simulink model "ACC_Test_module"  (R2017b)
settings: Solver=FixedStepAuto  StartTime=0.0  StopTime=150  FixedStep=0.05  RelTol=1e-3
libraries: simulink x4, SimOneModule x3
settings Model: Creator=weinan  LastModifiedBy=xuliang
settings SolverCC: AlgebraicLoopSolver=LineSearch

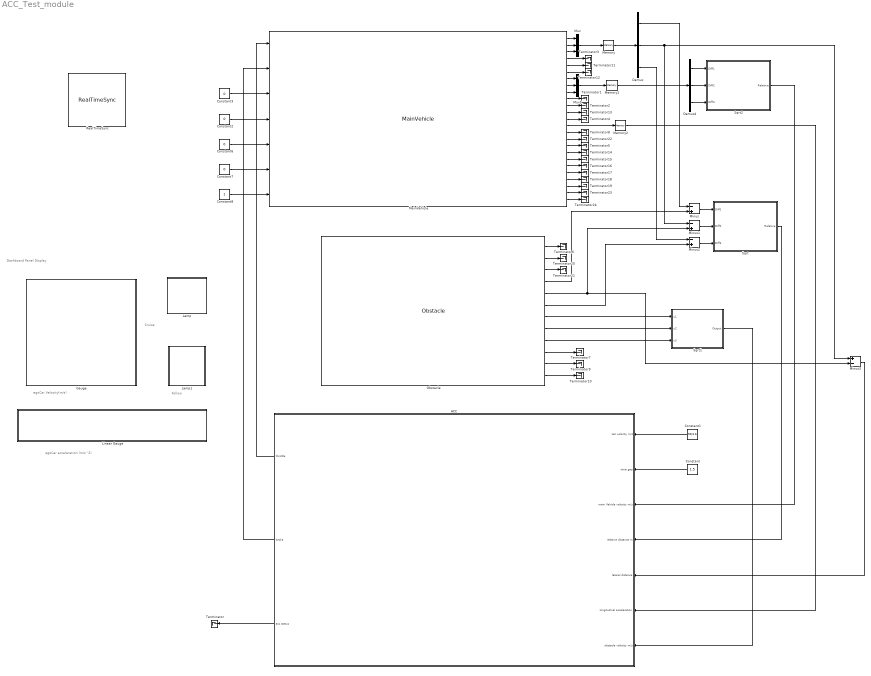
== system ACC_Test_module ==
  note: Cruise
  note: egoCar Velocity(m/s)
  note: Follow
  note: Dashboard Panel Display
  note: egoCar acceleration (m/s^2)
  "ACC " : Subsystem  mask(ACC){}
      mask help: ACC block
  Constant : Constant  Value=1.5  OutDataTypeStr=single
  Constant1 : Constant  Value=50/3.6  OutDataTypeStr=single
  Constant2 : Constant  Value=0  OutDataTypeStr=single
  Constant3 : Constant  Value=0  OutDataTypeStr=int32
  Constant6 : Constant  Value=0  OutDataTypeStr=boolean
  Constant7 : Constant  Value=0  OutDataTypeStr=boolean
  Constant8 : Constant  OutDataTypeStr=int32
  Demux : Demux  Outputs=3
  Demux4 : Demux  Outputs=3
  Gauge : Subsystem  DialogController=hmiCreateDDGDialog  IsWebBlock=on  mask(MWDashboardBlock){webBlockId=47d9afb7-ca15-4b52-9b06-8f3727cd5279, webBlockType=circulargauge, ShowInLibBrowser=on, ShowInitialText=on, HMISrcModelName=ACC_Test_module}
      mask prompts: webBlockId "WebBlock Id"; webBlockType "WebBlock Type"; HMISrcModelName "Source Model"
      mask help: SimulinkHMI:dialogs:CircularGaugeDialogDesc
      mask Help: helpview([docroot '/mapfiles/simulink.map'], 'hmi_gauge')
      mask Display:
      | if strcmp(get_param(bdroot(gcb),'BlockDiagramType'), 'library')
      |     image([(matlabroot) '/toolbox/simulink/hmi/icons/CircularGauge.png']);
      | end
  Lamp : Subsystem  DialogController=hmiCreateDDGDialog  IsWebBlock=on  mask(MWDashboardBlock){webBlockId=fddfa241-ada3-46a5-89fa-7b193cbd09ab, webBlockType=lamp, ShowInLibBrowser=on, ShowInitialText=on, HMISrcModelName=ACC_Test_module}
      mask prompts: webBlockId "WebBlock Id"; webBlockType "WebBlock Type"; HMISrcModelName "Source Model"
      mask help: Display a color that reflects an input value.
      mask Help: helpview([docroot '/mapfiles/simulink.map'], 'hmi_lamp')
      mask Display:
      | if strcmp(get_param(bdroot(gcb),'BlockDiagramType'),'library')
      |  image([(matlabroot) '/toolbox/simulink/hmi/icons/Lamp.png'])
      | end
  Lamp1 : Subsystem  DialogController=hmiCreateDDGDialog  IsWebBlock=on  mask(MWDashboardBlock){webBlockId=92ae66d2-b6c3-43d2-a72d-fb865ca14b34, webBlockType=lamp, ShowInLibBrowser=on, ShowInitialText=on, HMISrcModelName=ACC_Test_module}
      mask prompts: webBlockId "WebBlock Id"; webBlockType "WebBlock Type"; HMISrcModelName "Source Model"
      mask help: Display a color that reflects an input value.
      mask Help: helpview([docroot '/mapfiles/simulink.map'], 'hmi_lamp')
      mask Display:
      | if strcmp(get_param(bdroot(gcb),'BlockDiagramType'),'library')
      |  image([(matlabroot) '/toolbox/simulink/hmi/icons/Lamp.png'])
      | end
  Linear Gauge : Subsystem  DialogController=hmiCreateDDGDialog  IsWebBlock=on  mask(MWDashboardBlock){webBlockId=739a4254-edef-4805-a255-418ead3e1f6d, webBlockType=lineargauge, ShowInLibBrowser=on, ShowInitialText=on, HMISrcModelName=ACC_Test_module}
      mask prompts: webBlockId "WebBlock Id"; webBlockType "WebBlock Type"; HMISrcModelName "Source Model"
      mask help: SimulinkHMI:dialogs:LinearGaugeDialogDesc
      mask Help: helpview([docroot '/mapfiles/simulink.map'], 'hmi_linear_gauge')
      mask Display:
      | if strcmp(get_param(bdroot(gcb),'BlockDiagramType'), 'library')
      |     image([(matlabroot) '/toolbox/simulink/hmi/icons/LinearGauge.png']);
      | end
  MainVehicle : SimOneModule/MainVehicle
  Memory : Memory
  Memory1 : Memory
  Memory2 : Memory
  Minus : Sum  Inputs=-+
  Minus1 : Sum  Inputs=-+
  Minus2 : Sum  Inputs=-+
  Minus3 : Sum  Inputs=+-
  Mux : Mux  Inputs=3
  Mux1 : Mux  Inputs=3
  Obstacle : SimOneModule/Obstacle  MaxObstacleNum=10  ObstacleId=1
  RealTimeSync : SimOneModule/RealTimeSync
  "Sqrt " : Subsystem  mask(Sqrt){}
      mask help: Square root of the sum of squared inputs
  Sqrt1 : Subsystem  mask(Sqrt){}
      mask help: Square root of the sum of squared inputs
  Sqrt2 : Subsystem  mask(Sqrt){}
      mask help: Square root of the sum of squared inputs
  Terminator{,1..24} (25 alike) : Terminator
  wires:
  Constant8/1 -> MainVehicle/7
  Constant7/1 -> MainVehicle/6
  Constant6/1 -> MainVehicle/5
  Constant/1 -> "ACC "/2(time gap)
  Constant1/1 -> "ACC "/1(set velocity m/s)
  Mux/1 -> Memory/1
  "Sqrt "/1(Relative) -> "ACC "/4(relative distance m)
  Minus3/1 -> "ACC "/5(lateral distance)
  "ACC "/3(acc status) -> Terminator/1
  Memory/1 -> Demux/1
  Memory1/1 -> Demux4/1
  MainVehicle/11 -> Terminator2/1
  Minus/1 -> "Sqrt "/1(Diff1)
  Minus1/1 -> "Sqrt "/2(Diff2)
  Minus2/1 -> "Sqrt "/3(Diff3)
  Demux/1 -> Minus/1
  Demux/2 -> Minus3/1, Minus1/1
  Demux/3 -> Minus2/1
  Obstacle/4 -> Minus/2
  Obstacle/5 -> Minus3/2, Minus1/2
  Obstacle/6 -> Minus2/2
  Demux4/1 -> Sqrt2/1(Diff1)
  Demux4/2 -> Sqrt2/2(Diff2)
  Demux4/3 -> Sqrt2/3(Diff3)
  Sqrt2/1(Relative) -> "ACC "/3(main Vehicle velocity m/s)
  Sqrt1/1(Output) -> "ACC "/7(obstacle velocity m/s)
  Constant2/1 -> MainVehicle/4
  Memory2/1 -> "ACC "/6(longitudinal acceleration)
  MainVehicle/4 -> Terminator3/1
  Obstacle/10 -> Terminator7/1
  Obstacle/11 -> Terminator9/1
  Obstacle/12 -> Terminator10/1
  MainVehicle/2 -> Mux/2
  MainVehicle/1 -> Mux/1
  MainVehicle/3 -> Mux/3
  MainVehicle/5 -> Terminator11/1
  MainVehicle/6 -> Terminator12/1
  Mux1/1 -> Memory1/1
  MainVehicle/10 -> Terminator1/1
  MainVehicle/12 -> Terminator13/1
  MainVehicle/13 -> Terminator4/1
  MainVehicle/17 -> Terminator5/1
  MainVehicle/18 -> Terminator14/1
  MainVehicle/19 -> Terminator15/1
  MainVehicle/20 -> Terminator16/1
  MainVehicle/21 -> Terminator17/1
  MainVehicle/22 -> Terminator18/1
  MainVehicle/23 -> Terminator19/1
  Obstacle/1 -> Terminator6/1
  Obstacle/2 -> Terminator20/1
  Obstacle/3 -> Terminator21/1
  MainVehicle/14 -> Memory2/1
  MainVehicle/15 -> Terminator8/1
  MainVehicle/16 -> Terminator22/1
  "ACC "/1(throttle) -> MainVehicle/1
  "ACC "/2(brake) -> MainVehicle/2
  Obstacle/8 -> Sqrt1/2(u2)
  MainVehicle/8 -> Mux1/2
  Obstacle/9 -> Sqrt1/3(u3)
  MainVehicle/7 -> Mux1/1
  Obstacle/7 -> Sqrt1/1(u1)
  MainVehicle/9 -> Mux1/3
  MainVehicle/24 -> Terminator23/1
  MainVehicle/25 -> Terminator24/1
  Constant3/1 -> MainVehicle/3

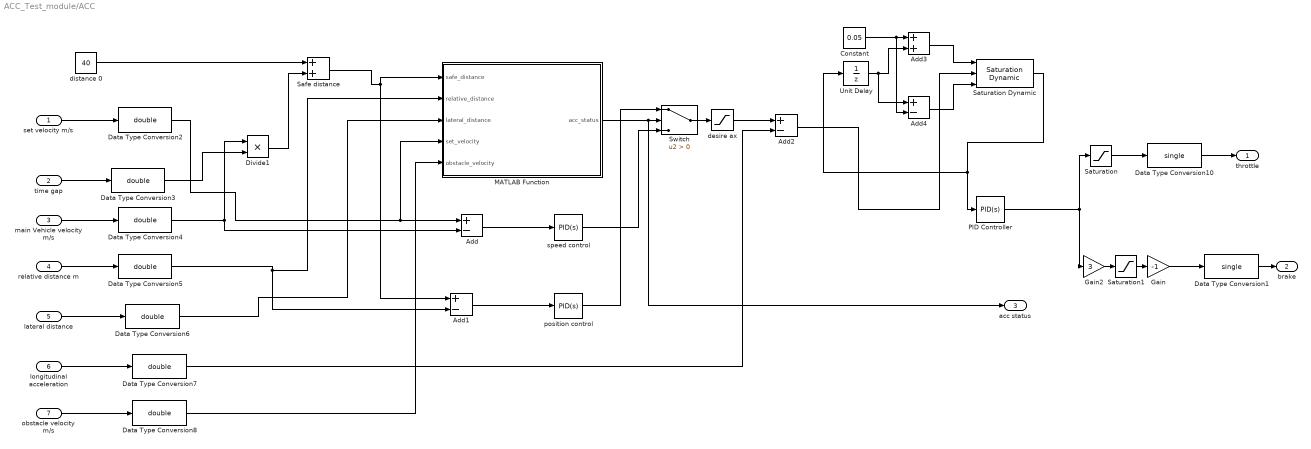
== system ACC_Test_module/ACC  ==
  set velocity m/s : Inport
  time gap : Inport  Port=2
  main Vehicle velocity m/s : Inport  Port=3
  relative distance m : Inport  Port=4
  lateral distance : Inport  Port=5
  longitudinal acceleration : Inport  Port=6
  obstacle velocity m/s : Inport  Port=7
  Add{,1..2,4} (4 alike) : Sum  Inputs=+-
  Add3 : Sum
  Constant : Constant  Value=0.05  OutDataTypeStr=double
  Data Type Conversion1 : DataTypeConversion  OutDataTypeStr=single
  Data Type Conversion10 : DataTypeConversion  OutDataTypeStr=single
  Data Type Conversion{2..8} (7 alike) : DataTypeConversion  OutDataTypeStr=double
  Divide1 : Product  Inputs=**
  Gain : Gain  Gain=-1
  Gain2 : Gain  Gain=3
  MATLAB Function : MATLAB Function  TreatAsAtomicUnit=on
  PID Controller : simulink/Continuous/PID Controller  Controller=PID  TimeDomain=Continuous-time  SampleTime=-1  IntegratorMethod=Forward Euler  FilterMethod=Forward Euler  Form=Parallel  UseFilter=on  ControllerParametersSource=internal  P=0.2  I=0  D=0  N=100  InitialConditionSource=internal  InitialConditionForIntegrator=0  InitialConditionForFilter=0  ExternalReset=none  LimitOutput=off  UpperSaturationLimit=inf  LowerSaturationLimit=-inf  LinearizeAsGain=on  AntiWindupMode=none  Kb=1  TrackingMode=off  Kt=1  PParamMin=[]  PParamMax=[]  IParamMin=[]  IParamMax=[]  DParamMin=[]  DParamMax=[]  NParamMin=[]  NParamMax=[]  KbParamMin=[]  KbParamMax=[]  KtParamMin=[]  KtParamMax=[]  POutMin=[]  POutMax=[]  IOutMin=[]  IOutMax=[]  DOutMin=[]  DOutMax=[]  NOutMin=[]  NOutMax=[]  KbOutMin=[]  KbOutMax=[]  KtOutMin=[]  KtOutMax=[]  IntegratorOutMin=[]  IntegratorOutMax=[]  FilterOutMin=[]  FilterOutMax=[]  SumOutMin=[]  SumOutMax=[]  SumI1OutMin=[]  SumI1OutMax=[]  SumI2OutMin=[]  SumI2OutMax=[]  SumI3OutMin=[]  SumI3OutMax=[]  SumDOutMin=[]  SumDOutMax=[]  SaturationOutMin=[]  SaturationOutMax=[]  IntegratorContinuousStateAttributes=''  IntegratorStateMustResolveToSignalObject=off  IntegratorRTWStateStorageClass=Auto  FilterContinuousStateAttributes=''  FilterStateMustResolveToSignalObject=off  FilterRTWStateStorageClass=Auto  DifferentiatorICPrevScaledInput=0  DifferentiatorOutMin=[]  DifferentiatorOutMax=[]  FilterDiffOutCoefMin=[]  FilterDiffOutCoefMax=[]  SumDenOutMin=[]  SumDenOutMax=[]  SumNumOutMin=[]  SumNumOutMax=[]  ReciprocalOutMin=[]  ReciprocalOutMax=[]  DivideOutMin=[]  DivideOutMax=[]  TunerSelectOption=Transfer Function Based (PID Tuner App)
  Safe distance : Sum
  Saturation : Saturate  UpperLimit=1  LowerLimit=0
  Saturation Dynamic : simulink/Discontinuities/Saturation Dynamic  OutMin=[]  OutMax=[]  OutDataTypeStr=Inherit: Same as second input  OutDataType=fixdt(1, 16)  OutScaling=2^-10  DoSatur=off
  Saturation1 : Saturate  UpperLimit=0  LowerLimit=-1
  Switch : Switch  Criteria=u2 > Threshold
  Unit Delay : UnitDelay  SampleTime=-1
  desire ax : Saturate  UpperLimit=8  LowerLimit=-3
  distance 0 : Constant  Value=40  OutDataTypeStr=double
  position control : simulink/Continuous/PID Controller  Controller=PID  TimeDomain=Continuous-time  SampleTime=-1  IntegratorMethod=Forward Euler  FilterMethod=Forward Euler  Form=Parallel  UseFilter=on  ControllerParametersSource=internal  P=-0.03  I=0  D=0  N=100  InitialConditionSource=internal  InitialConditionForIntegrator=0  InitialConditionForFilter=0  ExternalReset=none  LimitOutput=off  UpperSaturationLimit=inf  LowerSaturationLimit=-inf  LinearizeAsGain=on  AntiWindupMode=none  Kb=1  TrackingMode=off  Kt=1  PParamMin=[]  PParamMax=[]  IParamMin=[]  IParamMax=[]  DParamMin=[]  DParamMax=[]  NParamMin=[]  NParamMax=[]  KbParamMin=[]  KbParamMax=[]  KtParamMin=[]  KtParamMax=[]  POutMin=[]  POutMax=[]  IOutMin=[]  IOutMax=[]  DOutMin=[]  DOutMax=[]  NOutMin=[]  NOutMax=[]  KbOutMin=[]  KbOutMax=[]  KtOutMin=[]  KtOutMax=[]  IntegratorOutMin=[]  IntegratorOutMax=[]  FilterOutMin=[]  FilterOutMax=[]  SumOutMin=[]  SumOutMax=[]  SumI1OutMin=[]  SumI1OutMax=[]  SumI2OutMin=[]  SumI2OutMax=[]  SumI3OutMin=[]  SumI3OutMax=[]  SumDOutMin=[]  SumDOutMax=[]  SaturationOutMin=[]  SaturationOutMax=[]  IntegratorContinuousStateAttributes=''  IntegratorStateMustResolveToSignalObject=off  IntegratorRTWStateStorageClass=Auto  FilterContinuousStateAttributes=''  FilterStateMustResolveToSignalObject=off  FilterRTWStateStorageClass=Auto  DifferentiatorICPrevScaledInput=0  DifferentiatorOutMin=[]  DifferentiatorOutMax=[]  FilterDiffOutCoefMin=[]  FilterDiffOutCoefMax=[]  SumDenOutMin=[]  SumDenOutMax=[]  SumNumOutMin=[]  SumNumOutMax=[]  ReciprocalOutMin=[]  ReciprocalOutMax=[]  DivideOutMin=[]  DivideOutMax=[]  TunerSelectOption=Transfer Function Based (PID Tuner App)
  speed control : simulink/Continuous/PID Controller  Controller=PID  TimeDomain=Continuous-time  SampleTime=-1  IntegratorMethod=Forward Euler  FilterMethod=Forward Euler  Form=Parallel  UseFilter=on  ControllerParametersSource=internal  P=0.6  I=0  D=0  N=100  InitialConditionSource=internal  InitialConditionForIntegrator=0  InitialConditionForFilter=0  ExternalReset=none  LimitOutput=off  UpperSaturationLimit=inf  LowerSaturationLimit=-inf  LinearizeAsGain=on  AntiWindupMode=none  Kb=1  TrackingMode=off  Kt=1  PParamMin=[]  PParamMax=[]  IParamMin=[]  IParamMax=[]  DParamMin=[]  DParamMax=[]  NParamMin=[]  NParamMax=[]  KbParamMin=[]  KbParamMax=[]  KtParamMin=[]  KtParamMax=[]  POutMin=[]  POutMax=[]  IOutMin=[]  IOutMax=[]  DOutMin=[]  DOutMax=[]  NOutMin=[]  NOutMax=[]  KbOutMin=[]  KbOutMax=[]  KtOutMin=[]  KtOutMax=[]  IntegratorOutMin=[]  IntegratorOutMax=[]  FilterOutMin=[]  FilterOutMax=[]  SumOutMin=[]  SumOutMax=[]  SumI1OutMin=[]  SumI1OutMax=[]  SumI2OutMin=[]  SumI2OutMax=[]  SumI3OutMin=[]  SumI3OutMax=[]  SumDOutMin=[]  SumDOutMax=[]  SaturationOutMin=[]  SaturationOutMax=[]  IntegratorContinuousStateAttributes=''  IntegratorStateMustResolveToSignalObject=off  IntegratorRTWStateStorageClass=Auto  FilterContinuousStateAttributes=''  FilterStateMustResolveToSignalObject=off  FilterRTWStateStorageClass=Auto  DifferentiatorICPrevScaledInput=0  DifferentiatorOutMin=[]  DifferentiatorOutMax=[]  FilterDiffOutCoefMin=[]  FilterDiffOutCoefMax=[]  SumDenOutMin=[]  SumDenOutMax=[]  SumNumOutMin=[]  SumNumOutMax=[]  ReciprocalOutMin=[]  ReciprocalOutMax=[]  DivideOutMin=[]  DivideOutMax=[]  TunerSelectOption=Transfer Function Based (PID Tuner App)
  throttle : Outport
  brake : Outport  Port=2
  acc status : Outport  Port=3
  wires:
  time gap/1 -> Data Type Conversion3/1
  Divide1/1 -> Safe distance/2
  Safe distance/1 -> Add1/1, MATLAB Function/1(safe_distance)
  relative distance m/1 -> Data Type Conversion5/1
  lateral distance/1 -> Data Type Conversion6/1
  main Vehicle velocity m/s/1 -> Data Type Conversion4/1
  set velocity m/s/1 -> Data Type Conversion2/1
  Add/1 -> speed control/1
  obstacle velocity m/s/1 -> Data Type Conversion8/1
  Add1/1 -> position control/1
  speed control/1 -> Switch/3
  position control/1 -> Switch/1
  Switch/1 -> desire ax/1
  desire ax/1 -> Add2/1
  longitudinal acceleration/1 -> Data Type Conversion7/1
  Saturation/1 -> Data Type Conversion10/1
  Saturation1/1 -> Gain/1
  Gain/1 -> Data Type Conversion1/1
  Gain2/1 -> Saturation1/1
  Constant/1 -> Add4/2, Add3/1
  Unit Delay/1 -> Add4/1, Add3/2
  Add3/1 -> Saturation Dynamic/1
  Add4/1 -> Saturation Dynamic/3
  Add2/1 -> Saturation Dynamic/2
  Saturation Dynamic/1 -> Unit Delay/1, PID Controller/1
  PID Controller/1 -> Saturation/1, Gain2/1
  distance 0/1 -> Safe distance/1
  Data Type Conversion2/1 -> MATLAB Function/4(set_velocity), Add/1
  Data Type Conversion3/1 -> Divide1/2
  Data Type Conversion4/1 -> Add/2, Divide1/1
  Data Type Conversion5/1 -> Add1/2, MATLAB Function/2(relative_distance)
  Data Type Conversion6/1 -> MATLAB Function/3(lateral_distance)
  Data Type Conversion7/1 -> Add2/2
  Data Type Conversion8/1 -> MATLAB Function/5(obstacle_velocity)
  MATLAB Function/1(acc_status) -> acc status/1, Switch/2
  Data Type Conversion1/1 -> brake/1
  Data Type Conversion10/1 -> throttle/1

== system ACC_Test_module/Gauge ==

== system ACC_Test_module/Lamp ==

== system ACC_Test_module/Lamp1 ==

== system ACC_Test_module/Linear Gauge ==

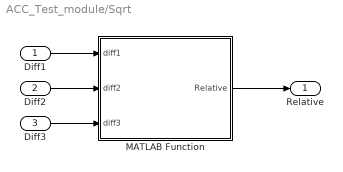
== system ACC_Test_module/Sqrt  ==
  Diff1 : Inport
  Diff2 : Inport  Port=2
  Diff3 : Inport  Port=3
  MATLAB Function : MATLAB Function  TreatAsAtomicUnit=on
  Relative : Outport
  wires:
  Diff1/1 -> MATLAB Function/1(diff1)
  MATLAB Function/1(Relative) -> Relative/1
  Diff2/1 -> MATLAB Function/2(diff2)
  Diff3/1 -> MATLAB Function/3(diff3)

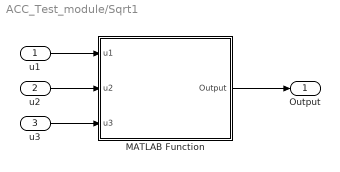
== system ACC_Test_module/Sqrt1 ==
  u1 : Inport
  u2 : Inport  Port=2
  u3 : Inport  Port=3
  MATLAB Function : MATLAB Function  TreatAsAtomicUnit=on
  Output : Outport
  wires:
  u1/1 -> MATLAB Function/1(u1)
  MATLAB Function/1(Output) -> Output/1
  u2/1 -> MATLAB Function/2(u2)
  u3/1 -> MATLAB Function/3(u3)

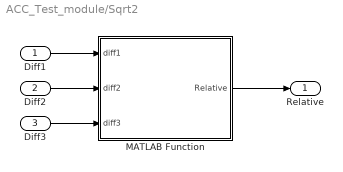
== system ACC_Test_module/Sqrt2 ==
  Diff1 : Inport
  Diff2 : Inport  Port=2
  Diff3 : Inport  Port=3
  MATLAB Function : MATLAB Function  TreatAsAtomicUnit=on
  Relative : Outport
  wires:
  Diff1/1 -> MATLAB Function/1(diff1)
  MATLAB Function/1(Relative) -> Relative/1
  Diff2/1 -> MATLAB Function/2(diff2)
  Diff3/1 -> MATLAB Function/3(diff3)

== matlab function ACC_Test_module/Sqrt2/MATLAB Function ==
  data: diff1 input; Relative output; diff2 input; diff3 input
function Relative = fcn(diff1,diff2,diff3)

Relative = sqrt(diff1 * diff1 + diff2 * diff2 + diff3 * diff3);

== matlab function ACC_Test_module/ACC /MATLAB Function ==
  data: safe_distance input; relative_distance input; lateral_distance input; acc_status output; set_velocity input; obstacle_velocity input
function acc_status = fcn(safe_distance,relative_distance,lateral_distance,set_velocity,obstacle_velocity)
acc_status=-1;   % default velocity control
if(abs(lateral_distance)<=1.75)   % front vehicle exists
    if(relative_distance<safe_distance && relative_distance>0 )
        acc_status=1;   % position control
    end
    if(set_velocity>obstacle_velocity)
        acc_status=1;   % position control
    end        
end

== matlab function ACC_Test_module/Sqrt /MATLAB Function ==
  data: diff1 input; Relative output; diff2 input; diff3 input
function Relative = fcn(diff1,diff2,diff3)

Relative = sqrt(diff1 * diff1 + diff2 * diff2 + diff3 * diff3);

== matlab function ACC_Test_module/Sqrt1/MATLAB Function ==
  data: u1 input; Output output; u2 input; u3 input
function Output = fcn(u1,u2,u3)

Output = sqrt(u1 * u1 + u2 * u2 + u3 * u3);
